simulink model "nowindupmodel"  (R2019a)
settings: Solver=VariableStepAuto  StartTime=0.0  StopTime=Tmax  RelTol=1e-3
values from neighbouring files (symbols this model uses):
  Kp = 5    [windup_test.m]    (also in workshop7.m = 2.66666666667)
  N = numel(Gall)    [ultgain.m]    (also in windup2_test.m = 10; windup_test.m = 10)
  Td = 0.8    [windup2_test.m]    (also in windup_test.m = 1)
  Ti = 7.5    [windup2_test.m]    (also in windup_test.m = 1; workshop7.m = 1.6)
settings Model: Creator=will  LastModifiedBy=will
settings DataIOCC: ReturnWorkspaceOutputs=off
settings DebuggingCC: PregeneratedLibrarySubsystemCodeDiagnostic=none  ArithmeticOperatorsInVariantConditions=warning
settings SFSimCC: SimUseLocalCustomCode=off
settings RTWCC: RTWUseLocalCustomCode=off

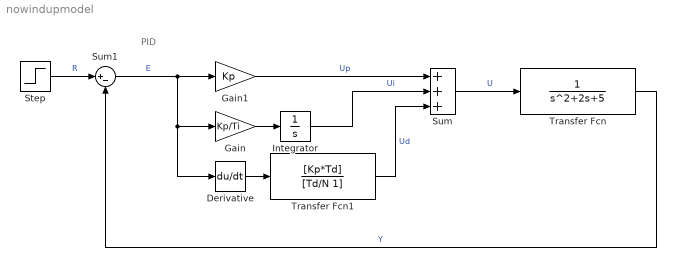
== system nowindupmodel ==
  note: PID
  Derivative : Derivative
  Gain : Gain  Gain=Kp/Ti
  Gain1 : Gain  Gain=Kp
  Integrator : Integrator
  Step : Step  SampleTime=0
  Sum : Sum  Inputs=+++
  Sum1 : Sum  Inputs=|+-
  Transfer Fcn : TransferFcn  Denominator=[1 2 5]
  Transfer Fcn1 : TransferFcn  Numerator=[Kp*Td]  Denominator=[Td/N 1]
  wires:
  Gain/1 -> Integrator/1
  Gain1/1 -> Sum/1  "Up"
  Integrator/1 -> Sum/2  "Ui"
  Transfer Fcn1/1 -> Sum/3  "Ud"
  Step/1 -> Sum1/1  "R"
  Transfer Fcn/1 -> Sum1/2  "Y"
  Sum1/1 -> Derivative/1, Gain/1, Gain1/1  "E"
  Sum/1 -> Transfer Fcn/1  "U"
  Derivative/1 -> Transfer Fcn1/1
